simulink model "Motor_Estimate"  (R2025a)
settings: Solver=VariableStepAuto  StartTime=0.0  StopTime=10.0  RelTol=1e-3
values from neighbouring files (symbols this model uses):
  motor_B = 1.036743055651295    (= 1.03674305565)    [Motor_Estimate_DataFile.m]    (also in control_system_designer.m = 0.78891; untitled.m = 0.78891)
  motor_J = 0.092718896322627    (= 0.0927188963226)    [Motor_Estimate_DataFile.m]    (also in control_system_designer.m = 0.029842; untitled.m = 0.029842)
  motor_Kt = 2.594477849336442    (= 2.59447784934)    [Motor_Estimate_DataFile.m]
  motor_L = 0.001741906    [Motor_Estimate_DataFile.m]    (also in control_system_designer.m; untitled.m)
  motor_n = 0.794535644305898    (= 0.794535644306)    [Motor_Estimate_DataFile.m]
  motor_R = 9.047391929    [Motor_Estimate_DataFile.m]    (also in control_system_designer.m; untitled.m)
settings Model: Creator=rajap  LastModifiedBy=rajap

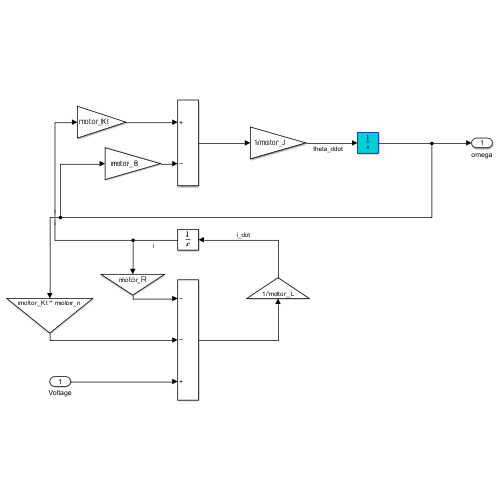
[thumbnail: Simulink's stored preview of the top-level diagram]
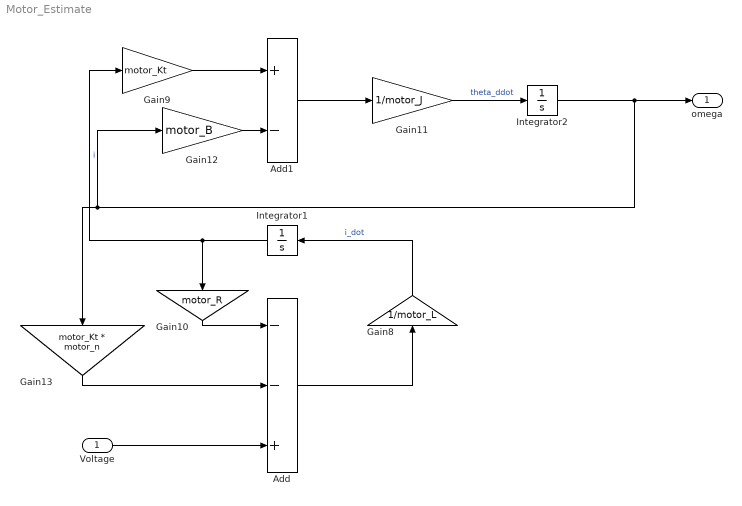
== system Motor_Estimate ==
  Voltage : Inport
  Add : Sum  Inputs=--+
  Add1 : Sum  Inputs=+-
  Gain10 : Gain  Gain=motor_R
  Gain11 : Gain  Gain=1/motor_J
  Gain12 : Gain  Gain=motor_B
  Gain13 : Gain  Gain=motor_Kt * motor_n
  Gain8 : Gain  Gain=1/motor_L
  Gain9 : Gain  Gain=motor_Kt
  Integrator1 : Integrator
  Integrator2 : Integrator
  omega : Outport
  wires:
  Integrator1/1 -> Gain10/1, Gain9/1  "i"
  Integrator2/1 -> omega/1, Gain13/1, Gain12/1
  Gain9/1 -> Add1/1
  Add/1 -> Gain8/1
  Gain10/1 -> Add/1
  Gain12/1 -> Add1/2
  Voltage/1 -> Add/3
  Add1/1 -> Gain11/1
  Gain13/1 -> Add/2
  Gain11/1 -> Integrator2/1  "theta_ddot"
  Gain8/1 -> Integrator1/1  "i_dot"
